simulink model "AeroECU"  (R2025a)
settings: Solver=FixedStepDiscrete  StartTime=0  StopTime=2  FixedStep=ecuTs  RelTol=1e-3
undefined symbols (not defined in the file): ecuTs
Description:
  | ARFWr RT ECU (Task 1.3). Reactive dual-wing law + hysteresis/dwell station snap at 100 Hz. In: SensorBus{vx,r,Tbrake,TbMax}. Out: ActuatorCmdBus, TvCmdBus (dTq=0 placeholder until T4.2). All law constants come from ecuLawParams(); ecuTs (sldd) owns FixedStep and the four Unit Delay rates.
settings Model: DataDictionary=ARFWr_RT.sldd  Creator=ASUS  LastModifiedBy=ASUS
settings DebuggingCC: InheritedTsInSrcMsg=error  TasksWithSamePriorityMsg=error  SigSpecEnsureSampleTimeMsg=error  UnknownTsInhSupMsg=error

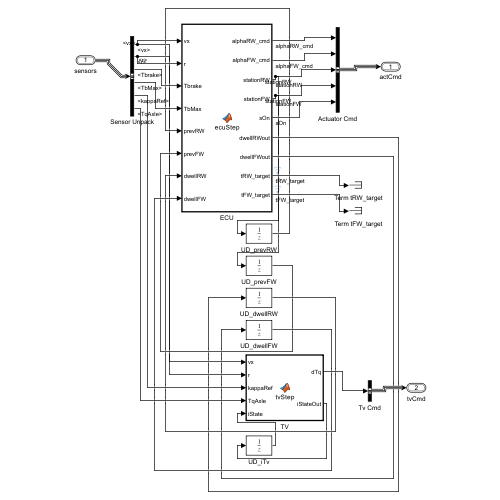
[thumbnail: Simulink's stored preview of the top-level diagram]
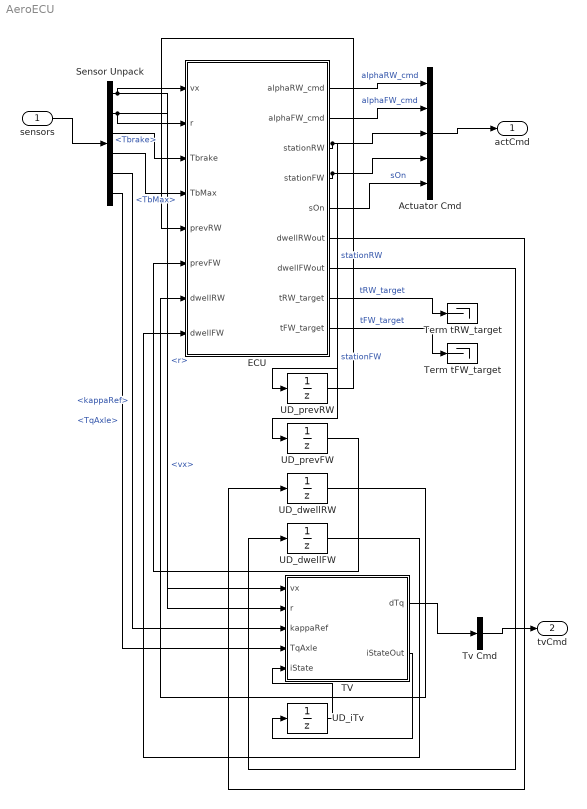
== system AeroECU ==
  sensors : Inport  OutDataTypeStr=Bus: SensorBus  PortDimensions=1  SampleTime=ecuTs
  Actuator Cmd : BusCreator  Inputs=5  OutDataTypeStr=Bus: ActuatorCmdBus
  ECU : MATLAB Function  TreatAsAtomicUnit=on
  Sensor Unpack : BusSelector  OutputSignals=vx,r,Tbrake,TbMax,kappaRef,TqAxle
  TV : MATLAB Function  TreatAsAtomicUnit=on
  Term tFW_target : Terminator
  Term tRW_target : Terminator
  Tv Cmd : BusCreator  Inputs=1  OutDataTypeStr=Bus: TvCmdBus
  UD_dwellFW : UnitDelay  SampleTime=ecuTs  HasFrameUpgradeWarning=on
  UD_dwellRW : UnitDelay  SampleTime=ecuTs  HasFrameUpgradeWarning=on
  UD_iTv : UnitDelay  Description=TV PI integrator state [Nm], closed outside the TV block. IC 0: the allocator starts with no accumulated yaw-rate error, matching simulink/validation/test_tvAlloc.m scenario 5 (zero error, zero state -> dTq == 0 exactly). Same Unit-Delay-outside-the-function pattern as UD_prevRW / UD_dwellRW.  SampleTime=ecuTs  HasFrameUpgradeWarning=on
  UD_prevFW : UnitDelay  InitialCondition=1  SampleTime=ecuTs  HasFrameUpgradeWarning=on
  UD_prevRW : UnitDelay  InitialCondition=1  SampleTime=ecuTs  HasFrameUpgradeWarning=on
  actCmd : Outport  OutDataTypeStr=Bus: ActuatorCmdBus
  tvCmd : Outport  Port=2  OutDataTypeStr=Bus: TvCmdBus
  wires:
  sensors/1 -> Sensor Unpack/1
  Sensor Unpack/1 -> ECU/1(vx), TV/1(vx)  "<vx>"
  Sensor Unpack/2 -> ECU/2(r), TV/2(r)  "<r>"
  Sensor Unpack/3 -> ECU/3(Tbrake)  "<Tbrake>"
  Sensor Unpack/4 -> ECU/4(TbMax)  "<TbMax>"
  UD_prevRW/1 -> ECU/5(prevRW)
  UD_prevFW/1 -> ECU/6(prevFW)
  UD_dwellRW/1 -> ECU/7(dwellRW)
  UD_dwellFW/1 -> ECU/8(dwellFW)
  ECU/1(alphaRW_cmd) -> Actuator Cmd/1  "alphaRW_cmd"
  ECU/2(alphaFW_cmd) -> Actuator Cmd/2  "alphaFW_cmd"
  ECU/3(stationRW) -> Actuator Cmd/3, UD_prevRW/1  "stationRW"
  ECU/4(stationFW) -> Actuator Cmd/4, UD_prevFW/1  "stationFW"
  ECU/5(sOn) -> Actuator Cmd/5  "sOn"
  ECU/6(dwellRWout) -> UD_dwellRW/1
  ECU/7(dwellFWout) -> UD_dwellFW/1
  Actuator Cmd/1 -> actCmd/1
  Tv Cmd/1 -> tvCmd/1
  Sensor Unpack/5 -> TV/3(kappaRef)  "<kappaRef>"
  Sensor Unpack/6 -> TV/4(TqAxle)  "<TqAxle>"
  UD_iTv/1 -> TV/5(iState)
  TV/2(iStateOut) -> UD_iTv/1
  TV/1(dTq) -> Tv Cmd/1
  ECU/8(tRW_target) -> Term tRW_target/1  "tRW_target"
  ECU/9(tFW_target) -> Term tFW_target/1  "tFW_target"

== matlab function AeroECU/TV ==
  data: vx input double; dTq output double; r input double; kappaRef input double; TqAxle input double; iState input double; iStateOut output double
function [dTq, iStateOut] = tvStep(vx, r, kappaRef, TqAxle, iState)
%#codegen
%TVSTEP  One ECU step of the front-axle torque-vectoring allocator.
%
%   Thin Simulink wrapper, exactly like the ECU block next to it: it calls the
%   review-verified reference function and does nothing else.
%     simulink/ecu/tvAllocStep.m   PI yaw-rate tracker + anti-windup + clamps
%     simulink/params/tvParams.m   gains, Ts, torque caps, enable switch
%
%   STATE. tvAllocStep is a pure function that RETURNS its updated integrator,
%   so the one state variable is closed OUTSIDE this block by a Unit Delay:
%       iStateOut -> UD_iTv -> iState     initial condition 0
%   Same pattern as stationRW -> UD_prevRW and dwellRWout -> UD_dwellRW.
%
%   PARAMETERS. tv comes from tvParams() called INSIDE the block, not from a
%   port: a MATLAB Function block cannot take a struct signal on an input port,
%   and tvParams is a no-input function whose fields are literals, so MATLAB
%   Coder constant-folds the whole call. Identical argument to the ECU block's
%   ecuLawParams() call, and it keeps tvParams.m the single source of truth
%   shared with simulink/validation/test_tvAlloc.m.
%
%   ENABLE. tv.enable is applied HERE and not inside tvAllocStep.m, so the
%   allocator itself stays a pure PI+clamp with no mode logic and gate T4.1's
%   five scenarios keep testing the allocator rather than a switch around it.
%   Both outputs are zeroed when disabled, so the integrator cannot accumulate
%   while bypassed. Being a constant-folded literal, this is a BUILD-TIME
%   switch: the generated ERT code contains either the allocator or a 0.
%
%   SIGNS (all checked against Scripts/vehModel.m, see tvAllocStep.m's header):
%   r > 0 and kappaRef > 0 are both LEFT; dTq > 0 sends MORE torque to the
%   RIGHT front wheel, which is a POSITIVE yaw moment (vehModel.m:697-698 sums
%   right-minus-left), i.e. it raises r toward kappaRef*vx. Plant/Torque Path's
%   torqueStep applies exactly TqAxle/2 -/+ dTq/2 on FL/FR, the same split
%   tvAllocStep.m's headroom clamp is derived from.

tv = tvParams();
if tv.enable > 0.5
    [dTq, iStateOut] = tvAllocStep(vx, r, kappaRef, TqAxle, iState, tv);
else
    dTq       = 0;
    iStateOut = 0;
end

end

== matlab function AeroECU/ECU ==
  data: vx input double; alphaRW_cmd output double; r input double; Tbrake input double; TbMax input double; prevRW input double; prevFW input double; dwellRW input double; dwellFW input double; alphaFW_cmd output double; stationRW output double; stationFW output double; sOn output double; dwellRWout output double; dwellFWout output double; tRW_target output double; tFW_target output double
function [alphaRW_cmd, alphaFW_cmd, stationRW, stationFW, sOn, dwellRWout, dwellFWout, ...
    tRW_target, tFW_target] = ...
    ecuStep(vx, r, Tbrake, TbMax, prevRW, prevFW, dwellRW, dwellFW)
%#codegen
%ECUSTEP  One ECU step of the ARFWr reactive dual-wing controller.
%
%   Thin Simulink wrapper: it calls the two review-verified reference
%   functions and does nothing else. It deliberately re-implements NOTHING.
%     simulink/ecu/ecuLawStep.m      continuous kappa/brake target
%     simulink/ecu/snapStationRef.m  hysteresis + minimum-dwell station snap
%
%   STATE. snapStationRef is a pure function that RETURNS its updated dwell
%   counters, so the four state variables are closed OUTSIDE this block by
%   four Unit Delays in AeroECU:
%       stationRW  -> UD_prevRW  -> prevRW    initial condition 1
%       stationFW  -> UD_prevFW  -> prevFW    initial condition 1
%       dwellRWout -> UD_dwellRW -> dwellRW   initial condition 0
%       dwellFWout -> UD_dwellFW -> dwellFW   initial condition 0
%   Those initial conditions reproduce the reference loop in
%   simulink/validation/test_snapRef.m EXACTLY (scenarios 1 and 3 both start
%   prevRW = prevFW = 1, dwellRW = dwellFW = 0). Consequence, by design: the
%   dwell test in snapStationRef is dwellCnt*Ts >= dwellMin, so with the
%   counter starting at 0 the first station switch cannot occur before
%   dwellMin = 0.2 s of simulated time. That startup lockout is the same one
%   the reference sequence tests exercise, and matching it is what makes the
%   Simulink ECU bit-identical to the desk reference for an identical input
%   sequence.
%
%   LAW CONSTANTS. law comes from ecuLawParams() called INSIDE the block, not
%   from a port and not from a duplicated set of Simulink.Parameter entries.
%   A MATLAB Function block cannot take a struct signal on an input port, and
%   ecuLawParams is a no-input function whose fields are literals, so MATLAB
%   Coder constant-folds the whole call: the generated ERT code contains the
%   numbers, not a struct or a function call. Keeping the call here means
%   ecuLawParams.m stays the single source of truth shared by this model, by
%   test_lawPort.m and by test_snapRef.m, which no snapshot in a data
%   dictionary could guarantee.
%
%   TbMax. The SensorBus carries TbMax, so the bus value is authoritative and
%   overrides the law default here. With the plant feeding the nominal
%   7000 Nm this is identical to the reference calls, which use
%   law.TbMax = 7000. TbMax must be strictly positive: ecuLawStep divides by
%   law.w1frac*law.TbMax. No guard is inserted, because a guard would be a
%   silent deviation from the ported formula.
%
%   SIGN. Tbrake is SIGNED, <= 0 when braking (same convention as
%   Scripts/vehModel.m and Functions/rwVelocityTarget.m). No abs().
%
%   sOn is passed through to snapStationRef only to keep the reference
%   signature; the snap decision does not use it, because tRW/tFW already
%   carry the brake overlay. sOn is published on ActuatorCmdBus for logging.
%   A value of sOn = 0.5 does NOT imply the brake station -- snapStationRef
%   is the single source of truth for which station is commanded.

law = ecuLawParams();
law.TbMax = TbMax;

[tRW, tFW, sOn] = ecuLawStep(vx, r, Tbrake, law);

[stIdxRW, stIdxFW, dwellRWout, dwellFWout] = snapStationRef( ...
    tRW, tFW, sOn, prevRW, prevFW, dwellRW, dwellFW, law);

stationRW = stIdxRW;
stationFW = stIdxFW;

% station index -> commanded angle [deg]. Done here rather than in a
% downstream lookup block so that law.stRW / law.stFW are read from the same
% ecuLawParams() call that produced the indices; a separate block would need
% its own copy of the station vectors and could drift out of step with it.
alphaRW_cmd = law.stRW(stIdxRW);
alphaFW_cmd = law.stFW(stIdxFW);

% T5.2 OBSERVABILITY ONLY. tRW/tFW are the CONTINUOUS pre-snap targets
% ecuLawStep already returned above; these two outputs publish them so the
% replay dashboard can draw the law target against the commanded staircase
% (simulink/viz/dashboardApp.m, logsout names tRW_target / tFW_target).
% They are pure copies -- nothing is recomputed and no control path reads
% them, so the ECU's behaviour is bit-identical with or without them. They
% are APPENDED to the signature so output ports 1-7 keep their numbering
% and AeroECU's root interface (actCmd / tvCmd) is unchanged.
tRW_target = tRW;
tFW_target = tFW;

end
